simulink model "RoboBoat_SScallv1"  (R2014a)
settings: Solver=FixedStepDiscrete  StartTime=0.0  StopTime=inf  FixedStep=.25  RelTol=1e-3
undefined symbols (not defined in the file): Com1, Com2, Com3, Com4, DiscIntNeverNeededParam, standard
libraries: xpcseriallib x31, visiontextngfix x25, simulink x19, slrtlib x9, speedgoatlib_IO102 x3, speedgoatlib x1
(part 4 of 5)

== system RoboBoat_SScallv1/Main FSM/Obstacle Navigation1/Obstacle Navigation/GPS: Bee Line/Approach ==
  Sensors : Inport
  RGB image : Inport  Port=2
  Enable : EnablePort
  Annotate Task : visiontextngfix/Insert Text  inputType=Obsolete  theText='GPS - Start: Approach - Distance: %f'  getTextLocFrom=Specify via dialog  textLoc=[10 70]  getTextColorFrom=Specify via dialog  textColor=[255 0 0]  getTextIntensityFrom=Specify via dialog  textIntensity=0  getTextOpacityFrom=Specify via dialog  textOpacity=1.0  dummyVar2=0  dummyVar3=0  dummyVar4=0  imagePorts=One multidimensional signal  isInputTransposed=off  fontFace=LucidaSansRegular  dummyVar1=0  blockFontSize=12  antiAliased=on
  Annotate Task2 : visiontextngfix/Insert Text  inputType=Obsolete  theText='Bee Line Approach'  getTextLocFrom=Specify via dialog  textLoc=[1 1]  getTextColorFrom=Specify via dialog  textColor=[0 0 0]  getTextIntensityFrom=Specify via dialog  textIntensity=0  getTextOpacityFrom=Specify via dialog  textOpacity=1.0  dummyVar2=0  dummyVar3=0  dummyVar4=0  imagePorts=One multidimensional signal  isInputTransposed=off  fontFace=LucidaSansRegular  dummyVar1=0  blockFontSize=12  antiAliased=on
  Annotate Task3 : visiontextngfix/Insert Text  inputType=Obsolete  theText='Obstacle- Distance: %f'  getTextLocFrom=Specify via dialog  textLoc=[10 100]  getTextColorFrom=Specify via dialog  textColor=[255 0 0]  getTextIntensityFrom=Specify via dialog  textIntensity=0  getTextOpacityFrom=Specify via dialog  textOpacity=1.0  dummyVar2=0  dummyVar3=0  dummyVar4=0  imagePorts=One multidimensional signal  isInputTransposed=off  fontFace=LucidaSansRegular  dummyVar1=0  blockFontSize=12  antiAliased=on
  Bus Selector : BusSelector  OutputSignals=Serial In.GPS.latitude,Serial In.GPS.longitude,Serial In.Buoy Info.Color ID,Serial In.Buoy Info.Distance
  Compare To Constant : simulink/Logic and Bit Operations/Compare To Constant  relop=<=  const=5  OutDataTypeStr=boolean
  Data Store Read : DataStoreRead  DataStoreName=obstNavEndGPS  SampleTime=0.1
  Data Type Conversion : DataTypeConversion  OutDataTypeStr=double
  Desired Heading and Distance : MATLAB Function  TreatAsAtomicUnit=on
  Obstacle Distance : MATLAB Function  TreatAsAtomicUnit=on
  Output Heirarchy : Subsystem
  Outputs : Outport
  Dodge Start : Outport  Port=2
  wires:
  Sensors/1 -> Output Heirarchy/3(Sensors), Bus Selector/1  "Sensors"
  Data Store Read/1 -> Desired Heading and Distance/1(DesiredGPS)
  Bus Selector/1 -> Desired Heading and Distance/2(GPSLat)  "<latitude>"
  Bus Selector/2 -> Desired Heading and Distance/3(GPSLong)  "<longitude>"
  Desired Heading and Distance/2(DesiredHeading) -> Output Heirarchy/2(Desired Heading)
  RGB image/1 -> Annotate Task2/1
  Desired Heading and Distance/1(Distance) -> Compare To Constant/1, Annotate Task/2
  Data Type Conversion/1 -> Output Heirarchy/1(Nav Finished)  "Task Finished"
  Output Heirarchy/1(Outputs) -> Outputs/1
  Annotate Task2/1 -> Annotate Task/1
  Annotate Task/1 -> Annotate Task3/1
  Annotate Task3/1 -> Output Heirarchy/4(Annotated Image)
  Obstacle Distance/2(DodgeStart) -> Dodge Start/1
  Compare To Constant/1 -> Data Type Conversion/1
  Obstacle Distance/1(ObstDist) -> Annotate Task3/2
  Bus Selector/3 -> Obstacle Distance/1(ColorID)  "<Color ID>"
  Bus Selector/4 -> Obstacle Distance/2(Dist)  "<Distance>"

== system RoboBoat_SScallv1/Main FSM/Obstacle Navigation1/Obstacle Navigation/GPS: Bee Line/Orient ==
  Sensors : Inport
  RGB image : Inport  Port=2
  Enable : EnablePort
  Annotate Task : visiontextngfix/Insert Text  inputType=Obsolete  theText='GPS - Center: Orient %f'  getTextLocFrom=Specify via dialog  textLoc=[10 70]  getTextColorFrom=Specify via dialog  textColor=[255 0 0]  getTextIntensityFrom=Specify via dialog  textIntensity=0  getTextOpacityFrom=Specify via dialog  textOpacity=1.0  dummyVar2=0  dummyVar3=0  dummyVar4=0  imagePorts=One multidimensional signal  isInputTransposed=off  fontFace=LucidaSansRegular  dummyVar1=0  blockFontSize=12  antiAliased=on
  Annotate Task1 : visiontextngfix/Insert Text  inputType=Obsolete  theText='Current Heading %f'  getTextLocFrom=Specify via dialog  textLoc=[10 40]  getTextColorFrom=Specify via dialog  textColor=[255 0 0]  getTextIntensityFrom=Specify via dialog  textIntensity=0  getTextOpacityFrom=Specify via dialog  textOpacity=1.0  dummyVar2=0  dummyVar3=0  dummyVar4=0  imagePorts=One multidimensional signal  isInputTransposed=off  fontFace=LucidaSansRegular  dummyVar1=0  blockFontSize=12  antiAliased=on
  Annotate Task2 : visiontextngfix/Insert Text  inputType=Obsolete  theText='Bee Line Orient'  getTextLocFrom=Specify via dialog  textLoc=[1 1]  getTextColorFrom=Specify via dialog  textColor=[0 0 0]  getTextIntensityFrom=Specify via dialog  textIntensity=0  getTextOpacityFrom=Specify via dialog  textOpacity=1.0  dummyVar2=0  dummyVar3=0  dummyVar4=0  imagePorts=One multidimensional signal  isInputTransposed=off  fontFace=LucidaSansRegular  dummyVar1=0  blockFontSize=12  antiAliased=on
  Bus Selector : BusSelector  OutputSignals=Serial In.GPS.latitude,Serial In.GPS.longitude,Serial In.Compass.Heading
  Data Store Read1 : DataStoreRead  DataStoreName=obstNavEndGPS  SampleTime=0.1
  Desired Heading : MATLAB Function  TreatAsAtomicUnit=on
  Output Heirarchy1 : Subsystem
  Within Range : MATLAB Function  TreatAsAtomicUnit=on
  Outputs : Outport
  Finished : Outport  Port=2
  wires:
  Sensors/1 -> Output Heirarchy1/3(Sensors), Bus Selector/1  "Sensors"
  Data Store Read1/1 -> Desired Heading/1(DesiredGPS)
  Bus Selector/1 -> Desired Heading/2(GPSLat)  "<latitude>"
  Bus Selector/2 -> Desired Heading/3(GPSLong)  "<longitude>"
  Desired Heading/1(DesiredHeading) -> Output Heirarchy1/2(Desired Heading), Annotate Task/2, Within Range/1(DesiredHeading)
  Bus Selector/3 -> Annotate Task1/2, Within Range/2(Compass)  "<Heading>"
  Within Range/1(Finished) -> Finished/1
  RGB image/1 -> Annotate Task2/1
  Output Heirarchy1/1(Outputs) -> Outputs/1
  Annotate Task/1 -> Annotate Task1/1
  Annotate Task1/1 -> Output Heirarchy1/1(Annotated Image)
  Annotate Task2/1 -> Annotate Task/1

== system RoboBoat_SScallv1/Main FSM/Start Speed/Gate Find and Through/Find/Output Heirarchy ==
  Sensors : Inport
  RPM : Inport  Port=2
  Desired Heading : Inport  Port=3
  Bus Creator{,1..2,4} (4 alike) : BusCreator  Inputs=2
  Bus Creator3 : BusCreator  Inputs=6
  C1 : Constant  Value=0  SampleTime=-1
  C2 : Constant  Value=0  SampleTime=-1
  C3 : Constant  Value=0  SampleTime=-1
  LPTask : Constant  SampleTime=-1
  Latitude : Constant  Value=0  SampleTime=-1
  Longitude : Constant  Value=0  SampleTime=-1
  Request Number : Constant  Value=0  SampleTime=-1
  Outputs : Outport
  wires:
  Bus Creator/1 -> Bus Creator1/1  "Control Signals"
  Bus Creator3/1 -> Bus Creator2/1  "Comms Panda"
  Request Number/1 -> Bus Creator3/1  "Request Number"
  Latitude/1 -> Bus Creator3/2  "Latitude"
  Longitude/1 -> Bus Creator3/3  "Longitude"
  C1/1 -> Bus Creator3/4  "C1"
  LPTask/1 -> Bus Creator2/2  "LIDAR Panda"
  Bus Creator1/1 -> Bus Creator4/1  "Outputs"
  Sensors/1 -> Bus Creator4/2  "Sensors"
  Bus Creator4/1 -> Outputs/1  "Output Signals"
  Bus Creator2/1 -> Bus Creator1/2  "Serial Outputs"
  C2/1 -> Bus Creator3/5  "C2"
  C3/1 -> Bus Creator3/6  "C3"
  RPM/1 -> Bus Creator/1  "RPM"
  Desired Heading/1 -> Bus Creator/2  "Desired Heading"

== system RoboBoat_SScallv1/Main FSM/Start Speed/Gate Find and Through/Through/Output Heirarchy ==
  Sensors : Inport
  RPM : Inport  Port=2
  Desired Heading : Inport  Port=3
  Bus Creator{,1..2,4} (4 alike) : BusCreator  Inputs=2
  Bus Creator3 : BusCreator  Inputs=6
  C1 : Constant  Value=0  SampleTime=-1
  C2 : Constant  Value=0  SampleTime=-1
  C3 : Constant  Value=0  SampleTime=-1
  LPTask : Constant  SampleTime=-1
  Latitude : Constant  Value=0  SampleTime=-1
  Longitude : Constant  Value=0  SampleTime=-1
  Request Number : Constant  Value=0  SampleTime=-1
  Outputs : Outport
  wires:
  Bus Creator/1 -> Bus Creator1/1  "Control Signals"
  Bus Creator3/1 -> Bus Creator2/1  "Comms Panda"
  Request Number/1 -> Bus Creator3/1  "Request Number"
  Latitude/1 -> Bus Creator3/2  "Latitude"
  Longitude/1 -> Bus Creator3/3  "Longitude"
  C1/1 -> Bus Creator3/4  "C1"
  LPTask/1 -> Bus Creator2/2  "LIDAR Panda"
  Bus Creator1/1 -> Bus Creator4/1  "Outputs"
  Sensors/1 -> Bus Creator4/2  "Sensors"
  Bus Creator4/1 -> Outputs/1  "Output Signals"
  Bus Creator2/1 -> Bus Creator1/2  "Serial Outputs"
  C2/1 -> Bus Creator3/5  "C2"
  C3/1 -> Bus Creator3/6  "C3"
  RPM/1 -> Bus Creator/1  "RPM"
  Desired Heading/1 -> Bus Creator/2  "Desired Heading"

== system RoboBoat_SScallv1/Main FSM/Start Speed/Gate Find and Through1/Find/Output Heirarchy ==
  Sensors : Inport
  RPM : Inport  Port=2
  Desired Heading : Inport  Port=3
  Bus Creator{,1..2,4} (4 alike) : BusCreator  Inputs=2
  Bus Creator3 : BusCreator  Inputs=6
  C1 : Constant  Value=0  SampleTime=-1
  C2 : Constant  Value=0  SampleTime=-1
  C3 : Constant  Value=0  SampleTime=-1
  LPTask : Constant  SampleTime=-1
  Latitude : Constant  Value=0  SampleTime=-1
  Longitude : Constant  Value=0  SampleTime=-1
  Request Number : Constant  Value=0  SampleTime=-1
  Outputs : Outport
  wires:
  Bus Creator/1 -> Bus Creator1/1  "Control Signals"
  Bus Creator3/1 -> Bus Creator2/1  "Comms Panda"
  Request Number/1 -> Bus Creator3/1  "Request Number"
  Latitude/1 -> Bus Creator3/2  "Latitude"
  Longitude/1 -> Bus Creator3/3  "Longitude"
  C1/1 -> Bus Creator3/4  "C1"
  LPTask/1 -> Bus Creator2/2  "LIDAR Panda"
  Bus Creator1/1 -> Bus Creator4/1  "Outputs"
  Sensors/1 -> Bus Creator4/2  "Sensors"
  Bus Creator4/1 -> Outputs/1  "Output Signals"
  Bus Creator2/1 -> Bus Creator1/2  "Serial Outputs"
  C2/1 -> Bus Creator3/5  "C2"
  C3/1 -> Bus Creator3/6  "C3"
  RPM/1 -> Bus Creator/1  "RPM"
  Desired Heading/1 -> Bus Creator/2  "Desired Heading"

== system RoboBoat_SScallv1/Main FSM/Start Speed/Gate Find and Through1/Through/Output Heirarchy ==
  Sensors : Inport
  RPM : Inport  Port=2
  Desired Heading : Inport  Port=3
  Bus Creator{,1..2,4} (4 alike) : BusCreator  Inputs=2
  Bus Creator3 : BusCreator  Inputs=6
  C1 : Constant  Value=0  SampleTime=-1
  C2 : Constant  Value=0  SampleTime=-1
  C3 : Constant  Value=0  SampleTime=-1
  LPTask : Constant  SampleTime=-1
  Latitude : Constant  Value=0  SampleTime=-1
  Longitude : Constant  Value=0  SampleTime=-1
  Request Number : Constant  Value=0  SampleTime=-1
  Outputs : Outport
  wires:
  Bus Creator/1 -> Bus Creator1/1  "Control Signals"
  Bus Creator3/1 -> Bus Creator2/1  "Comms Panda"
  Request Number/1 -> Bus Creator3/1  "Request Number"
  Latitude/1 -> Bus Creator3/2  "Latitude"
  Longitude/1 -> Bus Creator3/3  "Longitude"
  C1/1 -> Bus Creator3/4  "C1"
  LPTask/1 -> Bus Creator2/2  "LIDAR Panda"
  Bus Creator1/1 -> Bus Creator4/1  "Outputs"
  Sensors/1 -> Bus Creator4/2  "Sensors"
  Bus Creator4/1 -> Outputs/1  "Output Signals"
  Bus Creator2/1 -> Bus Creator1/2  "Serial Outputs"
  C2/1 -> Bus Creator3/5  "C2"
  C3/1 -> Bus Creator3/6  "C3"
  RPM/1 -> Bus Creator/1  "RPM"
  Desired Heading/1 -> Bus Creator/2  "Desired Heading"

== system RoboBoat_SScallv1/Sinks/actuators/analog output/Subsystem/Heading Controller ==
  Heading Desired : Inport
  Compass Heading : Inport  Port=2
  Gain : Gain  Gain=-0.05
  MATLAB Function : MATLAB Function  TreatAsAtomicUnit=on
  Saturation : Saturate  UpperLimit=5  LowerLimit=0
  Sum : Sum  Inputs=++|
  Voltage Nuetral : Constant  Value=2.5
  Steering : Outport
  wires:
  Compass Heading/1 -> MATLAB Function/2(CompassHeading)
  MATLAB Function/1(steering) -> Gain/1
  Gain/1 -> Sum/2
  Voltage Nuetral/1 -> Sum/1
  Sum/1 -> Saturation/1
  Saturation/1 -> Steering/1
  Heading Desired/1 -> MATLAB Function/1(HeadingDesired)

== system RoboBoat_SScallv1/Sinks/actuators/analog output/Subsystem/Propulsion Controller ==
  RPM : Inport
  Saturation : Saturate  UpperLimit=5  LowerLimit=0
  Sum : Sum  Inputs=++|
  Voltage Neutral : Constant  Value=2.5
  Volts / RPM : Gain  Gain=2.5/6000
  Propulsion : Outport
  wires:
  RPM/1 -> Volts / RPM/1
  Volts / RPM/1 -> Sum/2
  Voltage Neutral/1 -> Sum/1
  Sum/1 -> Saturation/1
  Saturation/1 -> Propulsion/1

== system RoboBoat_SScallv1/Sinks/actuators/analog output/Subsystem/data log ==
  Sensors signal : Inport
  Bus to Vector : BusToVector
  Scope 2 : slrtlib/Displays and Logging/Scope   scopeno=3  scopetype=File  autostart=on  viewmode=Graphical redraw  formatstr='%15.6f'  grid=on  ylimits=[0,0]  nosamples=250  noprepostsamples=0  interleave=1  triggermode=FreeRun  triggersignal=1  trigsignalfromport=off  triggerlevel=0.0  triggerslope=Either  triggerscope=1  triggersample=0  filename=Cmd_<%%%>.dat  mode=Commit  writesize=512  autorestart=on  dynamicfilemode=on  maxwritefilesize=512*1024^2
  wires:
  Sensors signal/1 -> Bus to Vector/1
  Bus to Vector/1 -> Scope 2/1

== system RoboBoat_SScallv1/Sinks/actuators/analog output/Subsystem/data log1 ==
  Sensors signal : Inport
  Bus to Vector : BusToVector
  Scope 2 : slrtlib/Displays and Logging/Scope   scopeno=4  scopetype=File  autostart=on  viewmode=Graphical redraw  formatstr='%15.6f'  grid=on  ylimits=[0,0]  nosamples=250  noprepostsamples=0  interleave=1  triggermode=FreeRun  triggersignal=1  trigsignalfromport=off  triggerlevel=0.0  triggerslope=Either  triggerscope=1  triggersample=0  filename=CoM_<%%%>.dat  mode=Commit  writesize=512  autorestart=on  dynamicfilemode=on  maxwritefilesize=512*1024^2
  wires:
  Sensors signal/1 -> Bus to Vector/1
  Bus to Vector/1 -> Scope 2/1

== system RoboBoat_SScallv1/Main FSM/Obstacle Navigation1/Obstacle Navigation/GPS: Bee Line/Approach/Output Heirarchy ==
  Nav Finished : Inport
  Desired Heading : Inport  Port=2
  Sensors : Inport  Port=3
  Annotated Image : Inport  Port=4
  Bus Creator : BusCreator  Inputs=3
  Bus Creator1 : BusCreator  Inputs=2
  Bus Creator2 : BusCreator  Inputs=3
  Bus Creator3 : BusCreator  Inputs=2
  Bus Creator4 : BusCreator  Inputs=2
  Due Sample Start : Constant  Value=0
  RPM Desired : Constant  Value=2000
  Ready to Read : Constant  Value=0
  Uno Power : Constant  Value=0
  Outputs : Outport
  wires:
  RPM Desired/1 -> Bus Creator/1  "RPM"
  Bus Creator/1 -> Bus Creator1/1  "Control Signals"
  Bus Creator2/1 -> Bus Creator/3  "Arduino Signals"
  Uno Power/1 -> Bus Creator2/2  "Uno Power"
  Desired Heading/1 -> Bus Creator/2  "Desired Heading"
  Bus Creator1/1 -> Bus Creator4/1  "Outputs"
  Annotated Image/1 -> Bus Creator1/2  "Annotated Image"
  Sensors/1 -> Bus Creator4/2  "Sensors"
  Bus Creator4/1 -> Bus Creator3/1  "Output Signals"
  Ready to Read/1 -> Bus Creator2/1  "Ready to Read"
  Due Sample Start/1 -> Bus Creator2/3  "Due Sample Start"
  Bus Creator3/1 -> Outputs/1
  Nav Finished/1 -> Bus Creator3/2  "Task Finished"

== system RoboBoat_SScallv1/Main FSM/Obstacle Navigation1/Obstacle Navigation/GPS: Bee Line/Orient/Output Heirarchy1 ==
  Annotated Image : Inport
  Desired Heading : Inport  Port=2
  Sensors : Inport  Port=3
  Bus Creator : BusCreator  Inputs=3
  Bus Creator1 : BusCreator  Inputs=2
  Bus Creator2 : BusCreator  Inputs=3
  Bus Creator3 : BusCreator  Inputs=2
  Bus Creator4 : BusCreator  Inputs=2
  Due Sample Start : Constant  Value=0
  Finished : Constant  Value=0
  RPM Desired : Constant  Value=0
  Ready to Read : Constant  Value=0
  Uno Power : Constant  Value=0
  Outputs : Outport
  wires:
  RPM Desired/1 -> Bus Creator/1  "RPM"
  Bus Creator/1 -> Bus Creator1/1  "Control Signals"
  Bus Creator2/1 -> Bus Creator/3  "Arduino Signals"
  Uno Power/1 -> Bus Creator2/2  "Uno Power"
  Desired Heading/1 -> Bus Creator/2  "Desired Heading"
  Bus Creator1/1 -> Bus Creator4/1  "Outputs"
  Annotated Image/1 -> Bus Creator1/2  "Annotated Image"
  Sensors/1 -> Bus Creator4/2  "Sensors"
  Bus Creator4/1 -> Bus Creator3/1  "Output Signals"
  Ready to Read/1 -> Bus Creator2/1  "Ready to Read"
  Due Sample Start/1 -> Bus Creator2/3  "Due Sample Start"
  Bus Creator3/1 -> Outputs/1
  Finished/1 -> Bus Creator3/2  "Task Finished"

== matlab function RoboBoat_SScallv1/Main FSM/Main Enabler ==
  data: taskSelector output; initEn output; ssGateEn output; RCEn output; RCHold input; initFin input; ssGateFin input; termEn output
function [taskSelector,initEn,ssGateEn,RCEn,termEn] = taskEnabler(RCHold,initFin,...
    ssGateFin)
%Written by Anderson Lebbad on July 19, 2013
%Last Edited: Edward Zhu on June 2, 2014
%   Substring search for task was written in
%   Case switches were redundant, combined with first set of if statements

%Changes the value of MainMode and the enablers for the tasks within the
%Main FSM.

% Initialize enable signals
RCEn = 0;
initEn = 0;
ssGateEn = 0;
termEn = 0;

% Set enable signals based on state completion
if initFin == 0
    initEn = 1;
    taskSelector = 1;
elseif RCHold == 0
    RCEn = 1;
    taskSelector = 3;
elseif ssGateFin == 0
    ssGateEn = 1;
    taskSelector = 2;
else
    termEn = 1;
    taskSelector = 4;
end

== matlab function RoboBoat_SScallv1/Sensors/Baseboard Serial/Compass Decode/Correct Heading Angle Magnetic to True North/Magnetic to True North Conversion ==
  data: HeadingM input; HeadingT output
function HeadingT = fcn(HeadingM)
% This block supports the Embedded MATLAB subset.
% See the help menu for details. 

HeadingT=HeadingM-12.3; %180 was added since compass was rotated when
                            %it was relocated.

if HeadingT>360
    HeadingT=HeadingT-360;
elseif HeadingT<0;
    HeadingT=HeadingT+360;
end

== matlab function RoboBoat_SScallv1/Main FSM/Obstacle Navigation1/Enter Gate/Gate 3 (White & Green)/MATLAB Function ==
  data: Prob input; RPM output; ColorID input; Dist input; Ang input; CurrentHeading input; GPSLat input; GPSLong input; Timer input; DesiredHeading output; gateGPS output
function [RPM,DesiredHeading,gateGPS] = navigation(Prob,ColorID,Dist,Ang,CurrentHeading,GPSLat,GPSLong,Timer)

% Function performs one buoy navigation through the start speed gates. If
% no buoys are found by the LIDAR/Vision assembly then an incremented
% turning algorithm is executed to turn by 10 degrees per increment up to 
% 90 degrees either way of the inital heading

% Written by Edward Zhu


persistent LockHeading TimeLastFound Counter Turn TurnInc gateLat gateLong

if isempty(LockHeading) && isempty(TimeLastFound) && isempty(Counter) && isempty(Turn) && isempty(TurnInc)
    LockHeading = CurrentHeading;
    TimeLastFound = 0;
    Counter = 0;
    TurnInc = 30;
    Turn = TurnInc;
    gateLat = 0;
    gateLong = 0;
end
Distance = Dist/100;
BoatWidth = 0.75;
Buffer = atan(2*BoatWidth/Distance);

WhiteOffset = Ang + Buffer;
GreenOffset = Ang - Buffer;

R = 6378137;

CurLat = (floor(GPSLat/100)+mod(GPSLat,100)/60)*pi/180;
CurLong = (ceil(GPSLong/100)-mod(-GPSLong,100)/60)*pi/180;

gateHeading = (mod(CurrentHeading - Ang, 360))*pi/180;

if ColorID == 2 && Prob > 0.9
    DesiredHeading = mod(LockHeading - Turn, 360);
    RPM = 0;
    GateFound = 1;
    TimeLastFound = Timer;
elseif ColorID == 3 && Prob > 0.9
    if Ang > 0
        DesiredHeading = mod(CurrentHeading - GreenOffset, 360);
    else
        DesiredHeading = mod(CurrentHeading + GreenOffset, 360);
    end
    RPM = 4000;
    GateFound = 1;
    TimeLastFound = Timer;
    gateLat =  asin(sin(CurLat)*cos(Distance/R) + cos(CurLat)*sin(Distance/R)*cos(gateHeading))*180/pi;
    gateLong = (CurLong + atan2(sin(gateHeading)*sin(Distance/R)*cos(CurLat),cos(Distance/R)-sin(CurLat)*sin(gateLat)))*180/pi;
else
    DesiredHeading = CurrentHeading;
    RPM = 0;
    GateFound = 0;
end

gateGPS = [gateLat gateLong];
TimeNoBuoys = Timer - TimeLastFound;

if GateFound == 0 && TimeNoBuoys > 15
    RPM = 0;
    DesiredHeading = mod(LockHeading - Turn, 360);
    HeadingDiff = DesiredHeading - CurrentHeading;
    gateGPS = [gateLat gateLong];
    
    if HeadingDiff > 180
        HeadingDiff = HeadingDiff - 360;
    elseif HeadingDiff < -180
        HeadingDiff = HeadingDiff + 360;
    end
    
    if HeadingDiff < 3
        Counter = Counter + 1;
    else
        Counter = 0;
    end
    
    if Counter >= 15
        Turn = Turn + TurnInc;
        Counter = 0;
        if abs(Turn) > 90
            TurnInc = -TurnInc;
        end
    end
end

== matlab function RoboBoat_SScallv1/Main FSM/Start Speed/GPS Enabler ==
  data: Finished input; SSMode output; Gate1 output; Gate2 output
function [SSMode, Gate1, Gate2] = GPSEnable(Finished)

%Written by Anderson Lebbad on June 9, 2015
%Last Edited: 
%
%This function enables Speedgate tasks. First the searches for and
%navigates through one gate, then the second.


%Parse Finished signal
OrientFinished = Finished(1);


%Initialize Enablers
Gate1 = 0;
Gate2 = 0;


%Switches the enable signal based on which task is flagged as done.
if OrientFinished == 0
    Gate1 = 1;
    SSMode = 1;
else
    Gate2 = 1;
    SSMode = 2;
end

== matlab function RoboBoat_SScallv1/Main FSM/Obstacle Navigation1/Exit Gate/Gate 1 (Red & White)/Distance ==
  data: Distance output; DesiredGPS input; GPSLat input; GPSLong input
function Distance  = DistCalc(DesiredGPS, GPSLat, GPSLong)

%Written by Anderson Lebbad on July 22, 2013
%Last Edited:

%Orients the boat towards a target GPS point before approaching it.
%This is done to keep the approach angle minimal, so the approach
%algorithm does not circle the target and never reach it.

%Parse input GPS and convert angles to radians
CurLat = (floor(GPSLat/100)+mod(GPSLat,100)/60)*pi/180;
CurLong = (floor(GPSLong/100)+mod(GPSLong,100)/60)*pi/180;
DesLat = (floor(DesiredGPS(1)/100)+mod(DesiredGPS(1),100)/60)*pi/180;
DesLong = (floor(DesiredGPS(2)/100)+mod(DesiredGPS(2),100)/60)*pi/180;
%Difference between lats and longs
DiffLat = DesLat - CurLat;
MidLat = cos((CurLat + DesLat)/2);
DiffLong = DesLong - CurLong;
%Radius of the earth in meters
R = 6378137;

%Calculate distance using the great-circle distance formula
%Formula documented here:
%   http://www.movable-type.co.uk/scripts/latlong.html
% a = sin(DiffLat/2)^2+sin(DiffLong/2)^2*cos(CurLat)*cos(DesLat);
% c = 2*atan2(sqrt(a), sqrt(1-a));
% Distance = R*c;

%Calculating distance using Pythagora's
a = DiffLong*MidLat;
b = DiffLat;
Distance = R*sqrt(a^2+b^2);

== matlab function RoboBoat_SScallv1/Main FSM/Obstacle Navigation1/Exit Gate/Gate 1 (Red & White)/MATLAB Function ==
  data: Prob input; RPM output; ColorID input; Dist input; Ang input; CurrentHeading input; GPSLat input; GPSLong input; Timer input; DesiredHeading output; gateGPS output
function [RPM,DesiredHeading,gateGPS] = navigation(Prob,ColorID,Dist,Ang,CurrentHeading,GPSLat,GPSLong,Timer)

% Function performs one buoy navigation through the start speed gates. If
% no buoys are found by the LIDAR/Vision assembly then an incremented
% turning algorithm is executed to turn by 10 degrees per increment up to 
% 90 degrees either way of the inital heading

% Written by Edward Zhu

persistent LockHeading TimeLastFound Counter Turn TurnInc gateLat gateLong

if isempty(LockHeading) && isempty(TimeLastFound) && isempty(Counter) && isempty(Turn) && isempty(TurnInc)
    LockHeading = CurrentHeading;
    TimeLastFound = 0;
    Counter = 0;
    TurnInc = 30;
    Turn = TurnInc;
    gateLat = 0;
    gateLong = 0;
end

Distance = Dist/100;

BoatWidth = 0.75;
Buffer = atan(2*BoatWidth/Distance);

RedOffset = Ang + Buffer;
WhiteOffset = Ang - Buffer;

R = 6378137;

CurLat = (floor(GPSLat/100)+mod(GPSLat,100)/60)*pi/180;
CurLong = (ceil(GPSLong/100)-mod(-GPSLong,100)/60)*pi/180;

gateHeading = (mod(CurrentHeading + Ang, 360))*pi/180;

if ColorID == 1 && Prob > 0.9
    if Ang < 0
        DesiredHeading = mod(CurrentHeading - RedOffset, 360);
    else
        DesiredHeading = mod(CurrentHeading + RedOffset, 360);
    end
    RPM = 4000;
    GateFound = 1;
    TimeLastFound = Timer;
    gateLat =  asin(sin(CurLat)*cos(Distance/R) + cos(CurLat)*sin(Distance/R)*cos(gateHeading))*180/pi;
    gateLong = (CurLong + atan2(sin(gateHeading)*sin(Distance/R)*cos(CurLat),cos(Distance/R)-sin(CurLat)*sin(gateLat)))*180/pi;
elseif ColorID == 2 && Prob > 0.9
    DesiredHeading = mod(LockHeading - Turn, 360);
    RPM = 0;
    GateFound = 1;
    TimeLastFound = Timer;
%     DesiredHeading = mod(CurrentHeading - WhiteOffset, 360);
%     RPM = 4000;
%     GateFound = 1;
%     TimeLastFound = Timer;
%     gateLat =  asin(sin(CurLat)*cos(Distance/R) + cos(CurLat)*sin(Distance/R)*cos(gateHeading))*180/pi;
%     gateLong = (CurLong + atan2(sin(gateHeading)*sin(Distance/R)*cos(CurLat),cos(Distance/R)-sin(CurLat)*sin(gateLat)))*180/pi;
else
    DesiredHeading = CurrentHeading;
    RPM = 0;
    GateFound = 0;
end

gateGPS = [gateLat gateLong];
TimeNoBuoys = Timer - TimeLastFound;

if GateFound == 0 && TimeNoBuoys > 15
    RPM = 0;
    DesiredHeading = mod(LockHeading - Turn, 360);
    HeadingDiff = DesiredHeading - CurrentHeading;
    gateGPS = [gateLat gateLong];
    
    if HeadingDiff > 180
        HeadingDiff = HeadingDiff - 360;
    elseif HeadingDiff < -180
        HeadingDiff = HeadingDiff + 360;
    end
    
    if HeadingDiff < 3
        Counter = Counter + 1;
    else
        Counter = 0;
    end
    
    if Counter >= 15
        Turn = Turn + TurnInc;
        Counter = 0;
        if abs(Turn) > 90
            TurnInc = -TurnInc;
        end
    end
end

== matlab function RoboBoat_SScallv1/Main FSM/Obstacle Navigation1/Exit Gate/Gate 2 (White & White)/Distance ==
  data: Distance output; DesiredGPS input; GPSLat input; GPSLong input
function Distance  = DistCalc(DesiredGPS, GPSLat, GPSLong)

%Written by Anderson Lebbad on July 22, 2013
%Last Edited:

%Orients the boat towards a target GPS point before approaching it.
%This is done to keep the approach angle minimal, so the approach
%algorithm does not circle the target and never reach it.

%Parse input GPS and convert angles to radians
CurLat = (floor(GPSLat/100)+mod(GPSLat,100)/60)*pi/180;
CurLong = (floor(GPSLong/100)+mod(GPSLong,100)/60)*pi/180;
DesLat = (floor(DesiredGPS(1)/100)+mod(DesiredGPS(1),100)/60)*pi/180;
DesLong = (floor(DesiredGPS(2)/100)+mod(DesiredGPS(2),100)/60)*pi/180;
%Difference between lats and longs
DiffLat = DesLat - CurLat;
MidLat = cos((CurLat + DesLat)/2);
DiffLong = DesLong - CurLong;
%Radius of the earth in meters
R = 6378137;

%Calculate distance using the great-circle distance formula
%Formula documented here:
%   http://www.movable-type.co.uk/scripts/latlong.html
% a = sin(DiffLat/2)^2+sin(DiffLong/2)^2*cos(CurLat)*cos(DesLat);
% c = 2*atan2(sqrt(a), sqrt(1-a));
% Distance = R*c;

%Calculating distance using Pythagora's
a = DiffLong*MidLat;
b = DiffLat;
Distance = R*sqrt(a^2+b^2);

== matlab function RoboBoat_SScallv1/Sensors/Baseboard Serial/GPS Decode/LLA to NED ==
  data: GPSLat input; GPSLong input; Lat output; Long output
function [Lat, Long] = LLA2NEDfun(GPSLat,GPSLong)
%Written by Anderson Lebbad on September 20, 2014
%Last edited by:
%
%This function converts the NMEA formatted GPS values to degrees for
%latitude and longitude.

Lat = (floor(GPSLat/100)+mod(GPSLat,100)/60);
%Negative added for being in western hemisphere
Long = -(ceil(GPSLong/100)-mod(-GPSLong,100)/60);

end

== matlab function RoboBoat_SScallv1/Main FSM/Obstacle Navigation1/Exit Gate/Gate 2 (White & White)/MATLAB Function ==
  data: Prob input; RPM output; ColorID input; Dist input; Ang input; CurrentHeading input; GPSLat input; GPSLong input; Timer input; DesiredHeading output; gateGPS output
function [RPM,DesiredHeading,gateGPS] = navigation(Prob,ColorID,Dist,Ang,CurrentHeading,GPSLat,GPSLong,Timer)

% Function performs one buoy navigation through the start speed gates. If
% no buoys are found by the LIDAR/Vision assembly then an incremented
% turning algorithm is executed to turn by 10 degrees per increment up to 
% 90 degrees either way of the inital heading

% Written by Edward Zhu


persistent LockHeading TimeLastFound Counter Turn TurnInc gateLat gateLong

if isempty(LockHeading) && isempty(TimeLastFound) && isempty(Counter) && isempty(Turn) && isempty(TurnInc)
    LockHeading = CurrentHeading;
    TimeLastFound = 0;
    Counter = 0;
    TurnInc = 30;
    Turn = TurnInc;
    gateLat = 0;
    gateLong = 0;
end
Distance = Dist/100;
BoatWidth = 0.75;
Buffer = atan(2*BoatWidth/Distance);

RedOffset = Ang + Buffer;
WhiteOffset = Ang - Buffer;

R = 6378137;

CurLat = (floor(GPSLat/100)+mod(GPSLat,100)/60)*pi/180;
CurLong = (ceil(GPSLong/100)-mod(-GPSLong,100)/60)*pi/180;

gateHeading = (mod(CurrentHeading - Ang, 360))*pi/180;

if ColorID == 1 && Prob > 0.9
    DesiredHeading = mod(CurrentHeading - RedOffset, 360);
    RPM = 2000;
    GateFound = 1;
    TimeLastFound = Timer;
    gateLat =  asin(sin(CurLat)*cos(Distance/R) + cos(CurLat)*sin(Distance/R)*cos(gateHeading))*180/pi;
    gateLong = (CurLong + atan2(sin(gateHeading)*sin(Distance/R)*cos(CurLat),cos(Distance/R)-sin(CurLat)*sin(gateLat)))*180/pi;
elseif ColorID == 2 && Prob > 0.9
    DesiredHeading = mod(CurrentHeading - WhiteOffset, 360);
    RPM = 2000;
    GateFound = 1;
    TimeLastFound = Timer;
    gateLat =  asin(sin(CurLat)*cos(Distance/R) + cos(CurLat)*sin(Distance/R)*cos(gateHeading))*180/pi;
    gateLong = (CurLong + atan2(sin(gateHeading)*sin(Distance/R)*cos(CurLat),cos(Distance/R)-sin(CurLat)*sin(gateLat)))*180/pi;
else
    DesiredHeading = CurrentHeading;
    RPM = 0;
    GateFound = 0;
end

gateGPS = [gateLat gateLong];
TimeNoBuoys = Timer - TimeLastFound;

if GateFound == 0 && TimeNoBuoys > 15
    RPM = 0;
    DesiredHeading = mod(LockHeading - Turn, 360);
    HeadingDiff = DesiredHeading - CurrentHeading;
    gateGPS = [gateLat gateLong];
    
    if HeadingDiff > 180
        HeadingDiff = HeadingDiff - 360;
    elseif HeadingDiff < -180
        HeadingDiff = HeadingDiff + 360;
    end
    
    if HeadingDiff < 3
        Counter = Counter + 1;
    else
        Counter = 0;
    end
    
    if Counter >= 15
        Turn = Turn + TurnInc;
        Counter = 0;
        if abs(Turn) > 90
            TurnInc = -TurnInc;
        end
    end
end

== matlab function RoboBoat_SScallv1/Main FSM/Obstacle Navigation1/Exit Gate/Gate 3 (White & Green)/Distance ==
  data: Distance output; DesiredGPS input; GPSLat input; GPSLong input
function Distance  = DistCalc(DesiredGPS, GPSLat, GPSLong)

%Written by Anderson Lebbad on July 22, 2013
%Last Edited:

%Orients the boat towards a target GPS point before approaching it.
%This is done to keep the approach angle minimal, so the approach
%algorithm does not circle the target and never reach it.

%Parse input GPS and convert angles to radians
CurLat = (floor(GPSLat/100)+mod(GPSLat,100)/60)*pi/180;
CurLong = (floor(GPSLong/100)+mod(GPSLong,100)/60)*pi/180;
DesLat = (floor(DesiredGPS(1)/100)+mod(DesiredGPS(1),100)/60)*pi/180;
DesLong = (floor(DesiredGPS(2)/100)+mod(DesiredGPS(2),100)/60)*pi/180;
%Difference between lats and longs
DiffLat = DesLat - CurLat;
MidLat = cos((CurLat + DesLat)/2);
DiffLong = DesLong - CurLong;
%Radius of the earth in meters
R = 6378137;

%Calculate distance using the great-circle distance formula
%Formula documented here:
%   http://www.movable-type.co.uk/scripts/latlong.html
% a = sin(DiffLat/2)^2+sin(DiffLong/2)^2*cos(CurLat)*cos(DesLat);
% c = 2*atan2(sqrt(a), sqrt(1-a));
% Distance = R*c;

%Calculating distance using Pythagora's
a = DiffLong*MidLat;
b = DiffLat;
Distance = R*sqrt(a^2+b^2);

== matlab function RoboBoat_SScallv1/Main FSM/Obstacle Navigation1/Exit Gate/Gate 3 (White & Green)/MATLAB Function ==
  data: Prob input; RPM output; ColorID input; Dist input; Ang input; CurrentHeading input; GPSLat input; GPSLong input; Timer input; DesiredHeading output; gateGPS output
function [RPM,DesiredHeading,gateGPS] = navigation(Prob,ColorID,Dist,Ang,CurrentHeading,GPSLat,GPSLong,Timer)

% Function performs one buoy navigation through the start speed gates. If
% no buoys are found by the LIDAR/Vision assembly then an incremented
% turning algorithm is executed to turn by 10 degrees per increment up to 
% 90 degrees either way of the inital heading

% Written by Edward Zhu


persistent LockHeading TimeLastFound Counter Turn TurnInc gateLat gateLong

if isempty(LockHeading) && isempty(TimeLastFound) && isempty(Counter) && isempty(Turn) && isempty(TurnInc)
    LockHeading = CurrentHeading;
    TimeLastFound = 0;
    Counter = 0;
    TurnInc = 30;
    Turn = TurnInc;
    gateLat = 0;
    gateLong = 0;
end
Distance = Dist/100;
BoatWidth = 0.75;
Buffer = atan(2*BoatWidth/Distance);

WhiteOffset = Ang + Buffer;
GreenOffset = Ang - Buffer;

R = 6378137;

CurLat = (floor(GPSLat/100)+mod(GPSLat,100)/60)*pi/180;
CurLong = (ceil(GPSLong/100)-mod(-GPSLong,100)/60)*pi/180;

gateHeading = (mod(CurrentHeading - Ang, 360))*pi/180;

if ColorID == 2 && Prob > 0.9
    DesiredHeading = mod(LockHeading - Turn, 360);
    RPM = 0;
    GateFound = 1;
    TimeLastFound = Timer;
elseif ColorID == 3 && Prob > 0.9
    if Ang > 0
        DesiredHeading = mod(CurrentHeading - GreenOffset, 360);
    else
        DesiredHeading = mod(CurrentHeading + GreenOffset, 360);
    end
    RPM = 4000;
    GateFound = 1;
    TimeLastFound = Timer;
    gateLat =  asin(sin(CurLat)*cos(Distance/R) + cos(CurLat)*sin(Distance/R)*cos(gateHeading))*180/pi;
    gateLong = (CurLong + atan2(sin(gateHeading)*sin(Distance/R)*cos(CurLat),cos(Distance/R)-sin(CurLat)*sin(gateLat)))*180/pi;
else
    DesiredHeading = CurrentHeading;
    RPM = 0;
    GateFound = 0;
end

gateGPS = [gateLat gateLong];
TimeNoBuoys = Timer - TimeLastFound;

if GateFound == 0 && TimeNoBuoys > 15
    RPM = 0;
    DesiredHeading = mod(LockHeading - Turn, 360);
    HeadingDiff = DesiredHeading - CurrentHeading;
    gateGPS = [gateLat gateLong];
    
    if HeadingDiff > 180
        HeadingDiff = HeadingDiff - 360;
    elseif HeadingDiff < -180
        HeadingDiff = HeadingDiff + 360;
    end
    
    if HeadingDiff < 3
        Counter = Counter + 1;
    else
        Counter = 0;
    end
    
    if Counter >= 15
        Turn = Turn + TurnInc;
        Counter = 0;
        if abs(Turn) > 90
            TurnInc = -TurnInc;
        end
    end
end

== matlab function RoboBoat_SScallv1/Main FSM/Obstacle Navigation1/Exit Gate/MATLAB Function ==
  data: gateID input; outputSelector output; gate1En output; gate2En output; gate3En output
function [outputSelector,gate1En,gate2En,gate3En] = gateSelector(gateID)
% Determines which colors to filter for based on the gateID as received
% from the judges

gate1En = 0;
gate2En = 0;
gate3En = 0;

if gateID == 1
    gate1En = 1;
    outputSelector = 1;
elseif gateID == 2
    gate2En = 1;
    outputSelector = 2;
else
    gate3En = 1;
    outputSelector = 3;
end

== matlab function RoboBoat_SScallv1/Main FSM/Start Speed/Gate Find and Through/Find/MATLAB Function1 ==
  data: Dist input; Angles input; X input; Y input; Heading input; found output; Goal output; DesiredHeading output
function [found, Goal, DesiredHeading] = SpeedGate(Dist,Angles,X,Y,Heading)
%Written by Anderson Lebbad on May 29, 2015
%Last Edited by:

%This function sends theboat forward until a landmark is found, then it
%navigates towards the right of it.

persistent goalX goalY Found initialHeading change
if isempty(goalX)
    goalX = X;
    goalY = Y;
    Found = 0;
    initialHeading = Heading;
    change = 10;
end

DesiredHeading = Heading;
DistM = Dist./100;
dodgeWidth = 3;

if Found == 0
    if DistM(2) ~= 0
        %If two objects are found, set goal between the two
        w = (DistM(1)*sin(Angles(1)) + DistM(2)*sin(Angles(2)*pi/180)) / 2;
        h = (DistM(1)*cos(Angles(1)) + DistM(2)*sin(Angles(2)*pi/180)) / 2;
        goalX = X + h*cos(Heading) - w*sin(Heading);
        goalY = Y + h*sin(Heading) + w*cos(Heading);
        Found = 1;
    elseif DistM(1) ~= 0
        %If one object is found, set goal dodgewidth to the right of it
        w = DistM(1)*sin(Angles(1)) + dodgeWidth;
        h = DistM(1)*cos(Angles(1));
        goalX = X + h*cos(Heading) - w*sin(Heading);
        goalY = Y + h*sin(Heading) + w*cos(Heading);
        Found = 1;
    else
        %If no objects are found, search. Scan 30 degrees to left and right
        %of initial heading.
        DesiredHeading = Heading + change;
        if abs(DesiredHeading - initialHeading) > 30
            change = -change;
            DesiredHeading = Heading + change;
        end
    end
end

Goal = [goalX, goalY];
found = Found;

end

== matlab function RoboBoat_SScallv1/Main FSM/Obstacle Navigation1/Enter Gate/Gate 1 (Red & White)/MATLAB Function ==
  data: Prob input; RPM output; ColorID input; Dist input; Ang input; CurrentHeading input; GPSLat input; GPSLong input; Timer input; DesiredHeading output; gateGPS output
function [RPM,DesiredHeading,gateGPS] = navigation(Prob,ColorID,Dist,Ang,CurrentHeading,GPSLat,GPSLong,Timer)

% Function performs one buoy navigation through the start speed gates. If
% no buoys are found by the LIDAR/Vision assembly then an incremented
% turning algorithm is executed to turn by 10 degrees per increment up to 
% 90 degrees either way of the inital heading

% Written by Edward Zhu

persistent LockHeading TimeLastFound Counter Turn TurnInc gateLat gateLong

if isempty(LockHeading) && isempty(TimeLastFound) && isempty(Counter) && isempty(Turn) && isempty(TurnInc)
    LockHeading = CurrentHeading;
    TimeLastFound = 0;
    Counter = 0;
    TurnInc = 30;
    Turn = TurnInc;
    gateLat = 0;
    gateLong = 0;
end

Distance = Dist/100;

BoatWidth = 0.75;
Buffer = atan(2*BoatWidth/Distance);

RedOffset = Ang + Buffer;
WhiteOffset = Ang - Buffer;

R = 6378137;

CurLat = (floor(GPSLat/100)+mod(GPSLat,100)/60)*pi/180;
CurLong = (ceil(GPSLong/100)-mod(-GPSLong,100)/60)*pi/180;

gateHeading = (mod(CurrentHeading + Ang, 360))*pi/180;

if ColorID == 1 && Prob > 0.9
    if Ang < 0
        DesiredHeading = mod(CurrentHeading - RedOffset, 360);
    else
        DesiredHeading = mod(CurrentHeading + RedOffset, 360);
    end
    RPM = 4000;
    GateFound = 1;
    TimeLastFound = Timer;
    gateLat =  asin(sin(CurLat)*cos(Distance/R) + cos(CurLat)*sin(Distance/R)*cos(gateHeading))*180/pi;
    gateLong = (CurLong + atan2(sin(gateHeading)*sin(Distance/R)*cos(CurLat),cos(Distance/R)-sin(CurLat)*sin(gateLat)))*180/pi;
elseif ColorID == 2 && Prob > 0.9
    DesiredHeading = mod(LockHeading - Turn, 360);
    RPM = 0;
    GateFound = 1;
    TimeLastFound = Timer;
%     DesiredHeading = mod(CurrentHeading - WhiteOffset, 360);
%     RPM = 4000;
%     GateFound = 1;
%     TimeLastFound = Timer;
%     gateLat =  asin(sin(CurLat)*cos(Distance/R) + cos(CurLat)*sin(Distance/R)*cos(gateHeading))*180/pi;
%     gateLong = (CurLong + atan2(sin(gateHeading)*sin(Distance/R)*cos(CurLat),cos(Distance/R)-sin(CurLat)*sin(gateLat)))*180/pi;
else
    DesiredHeading = CurrentHeading;
    RPM = 0;
    GateFound = 0;
end

gateGPS = [gateLat gateLong];
TimeNoBuoys = Timer - TimeLastFound;

if GateFound == 0 && TimeNoBuoys > 15
    RPM = 0;
    DesiredHeading = mod(LockHeading - Turn, 360);
    HeadingDiff = DesiredHeading - CurrentHeading;
    gateGPS = [gateLat gateLong];
    
    if HeadingDiff > 180
        HeadingDiff = HeadingDiff - 360;
    elseif HeadingDiff < -180
        HeadingDiff = HeadingDiff + 360;
    end
    
    if HeadingDiff < 3
        Counter = Counter + 1;
    else
        Counter = 0;
    end
    
    if Counter >= 15
        Turn = Turn + TurnInc;
        Counter = 0;
        if abs(Turn) > 90
            TurnInc = -TurnInc;
        end
    end
end

== matlab function RoboBoat_SScallv1/Main FSM/Start Speed/Gate Find and Through1/GPS Enabler ==
  data: Finished input; GPSMode output; OrientEn output; ApproachEn output
function [GPSMode, OrientEn, ApproachEn] = GPSEnable(Finished)

%Written by Anderson Lebbad on July 22, 2013
%Last Edited: July 27, 2013
%   Removed Termination Block

%This function enables GPS tasks. First the boat orients towards the
%target, then it approaches it.


%Parse Finished signal
OrientFinished = Finished(1);


%Initialize Enablers
OrientEn = 0;
ApproachEn = 0;


%Switches the enable signal based on which task is flagged as done.
if OrientFinished == 0
    OrientEn = 1;
    GPSMode = 1;
else
    ApproachEn = 1;
    GPSMode = 2;
end

== matlab function RoboBoat_SScallv1/Main FSM/Obstacle Navigation1/Enter Gate/MATLAB Function ==
  data: gateID input; outputSelector output; gate1En output; gate2En output; gate3En output
function [outputSelector,gate1En,gate2En,gate3En] = gateSelector(gateID)
% Determines which colors to filter for based on the gateID as received
% from the judges

gate1En = 0;
gate2En = 0;
gate3En = 0;

if gateID == 1
    gate1En = 1;
    outputSelector = 1;
elseif gateID == 2
    gate2En = 1;
    outputSelector = 2;
else
    gate3En = 1;
    outputSelector = 3;
end

== matlab function RoboBoat_SScallv1/Main FSM/Obstacle Navigation1/Obstacle Navigation/MATLAB Function ==
  data: dodgeIncomplete input; dodgeStart input; taskSelector output; dodgeEn output; GPSEn output
function [taskSelector, dodgeEn, GPSEn]  = obstNavEnabler(dodgeIncomplete, dodgeStart)

GPSEn = 0;
dodgeEn = 0;

if  dodgeStart == 1 || dodgeIncomplete == 1
    dodgeEn = 1;
    taskSelector = 1;
else
    GPSEn = 1;
    taskSelector = 2;
end

== matlab function RoboBoat_SScallv1/Main FSM/Obstacle Navigation1/Task Option1/Message Composer ==
  data: taskStrInit input; taskStrAdj output
function taskStrAdj = composeMessage(taskStrInit)
%Written by Anderson Lebbad on August 9, 2013
%Last Edited: Edward Zhu on June 2, 2014

%This function adjusts the length of a vector to a set value by filling
%the remaining space with 0's. This is necessary for data store objects
%that have a fixed size for the memory allocation, but a variable length
%input.

%Length of message packet
strLength = 8;

%Size of text in message
taskStrLength = size(taskStrInit,1);

%Pad end of text with zeros
taskStrAdj = [taskStrInit' zeros(1,strLength-taskStrLength)];

== matlab function RoboBoat_SScallv1/Main FSM/Obstacle Navigation1/GPS: Center/Orient/Desired Heading ==
  data: DesiredGPS input; DesiredHeading output; GPSLat input; GPSLong input
function DesiredHeading = Orient(DesiredGPS, GPSLat, GPSLong)

%Written by Anderson Lebbad on July 22, 2013
%Last Edited: Edward Zhu on July 5, 2014

% Edit:
% Changed calculation to use positive lat and negative long

%Orients the boat towards a target GPS point before approaching it.
%This is done to keep the approach angle minimal, so the approach
%algorithm does not circle the target and never reach it.

%Parse input GPS and convert angles to radians
CurLat = (floor(GPSLat/100)+mod(GPSLat,100)/60)*pi/180;
CurLong = (ceil(GPSLong/100)-mod(-GPSLong,100)/60)*pi/180;
DesLat = (floor(DesiredGPS(1)/100)+mod(DesiredGPS(1),100)/60)*pi/180;
DesLong = (ceil(DesiredGPS(2)/100)-mod(-DesiredGPS(2),100)/60)*pi/180;

%Difference between longs
DiffLong = DesLong - CurLong;

%Calculate initial bearing - formula documented here: 
%   http://www.movable-type.co.uk/scripts/latlong.html
y = sin(DiffLong)*cos(DesLat);
x = cos(CurLat)*sin(DesLat)-sin(CurLat)*cos(DesLat)*cos(DiffLong);
DesiredHeading = mod(atan2(y, x)*180/pi + 360, 360);

== matlab function RoboBoat_SScallv1/Main FSM/Obstacle Navigation1/MATLAB Function1 ==
  data: taskMode input; taskSelector output; startGPSFin input; commFin input; enterGateFin input; obstNavFin input; startGPSEn output; commEn output; enterGateEn output; obstNavEn output; exitGateEn output
function [taskSelector,startGPSEn,commEn,enterGateEn,obstNavEn,exitGateEn]...
    = taskEnabler(taskMode,startGPSFin,commFin,enterGateFin,obstNavFin)

startGPSEn = 0;
commEn = 0;
enterGateEn = 0;
obstNavEn = 0;
exitGateEn = 0;

taskOption = char(taskMode);

if ~isempty(strfind(taskOption,'Comm'))
    startGPSFin = 1;
elseif ~isempty(strfind(taskOption,'Enter'))
    startGPSFin = 1;
    commFin = 1;
elseif ~isempty(strfind(taskOption,'Nav'))
    startGPSFin = 1;
    commFin = 1;
    enterGateFin = 1;
elseif ~isempty(strfind(taskOption,'Exit'))
    startGPSFin = 1;
    commFin = 1;
    enterGateFin = 1;
    obstNavFin = 1;
end

if startGPSFin == 0
    startGPSEn = 1;
    taskSelector = 1;
elseif commFin == 0
    commEn = 1;
    taskSelector = 2;
elseif enterGateFin == 0
    enterGateEn = 1;
    taskSelector = 3;
elseif obstNavFin == 0
    obstNavEn = 1;
    taskSelector = 4;
else
    exitGateEn = 1;
    taskSelector = 5;
end

== matlab function RoboBoat_SScallv1/Main FSM/Obstacle Navigation1/Obstacle Navigation/GPS: Bee Line/Approach/Obstacle Distance ==
  data: ColorID input; ObstDist output; DodgeStart output; Dist input
function [ObstDist, DodgeStart] = obstDist(ColorID,Dist)

%Written by Edward Zhu
%Last Edited by:

ObstDist = Dist / 100;

% if ColorID == 5 || ColorID == 6
    if ObstDist <= 3
        DodgeStart = 1;
    else
        DodgeStart = 0;
    end
% else
%     DodgeStart = 0;
% end

== matlab function RoboBoat_SScallv1/Main FSM/Obstacle Navigation1/Obstacle Navigation/GPS: Bee Line/GPS Enabler ==
  data: Finished input; GPSMode output; OrientEnable output; ApproachEnable output
function [GPSMode, OrientEnable, ApproachEnable] =...
    GPSEnable(Finished)

%Written by Anderson Lebbad on July 22, 2013
%Last Edited: July 27, 2013
%   Removed Termination Block

%This function enables GPS tasks. First the boat orients towards the
%target, then it approaches it.


%Parse Finished signal
OrientFinished = Finished(1);


%Initialize Enablers
OrientEnable = 0;
ApproachEnable = 0;


%Switches the enable signal based on which task is flagged as done.
if OrientFinished == 0
    OrientEnable = 1;
    GPSMode = 1;
else
    ApproachEnable = 1;
    GPSMode = 2;
end
